simulink model "pfb_fir_2p_2kpt_12i_18o_os2_core"  (R2021a)
(part 3 of 41)

      mask prompts: mult_latency "Multiplier Latency"; coeff_width "Coefficient Bit Width In"; coeff_frac_width "Coefficient Fractional Bits"; delay "Data/Sync Delay"; data_width "Data Bit Width In"; bram_latency "BRAM Latency"; use_hdl "Use behavioral HDL for multlipliers"; use_embedded "Use embedded multipliers"
      mask init: same as pfb_fir_2p_2kpt_12i_18o_os2_core/pfb_fir/pol1_in10_tap2
      mask Callback use_hdl:
      | use_hdl = get_param(gcb,'use_hdl');
      | if( strcmp(use_hdl,'on')),
      |     set_param(gcb, 'use_embedded','off');
      |     set_param(gcb, 'MaskVisibilities',{'on','on','on','on','on','on','on','off'});
      | else,
      |     set_param(gcb, 'MaskVisibilities',{'on','on','on','on','on','on','on','on'});
      | end
  pol1_in8_tap3 : Subsystem  AncestorBlock=casper_library_pfbs/tap  mask(tap){mult_latency=2, coeff_width=18, coeff_frac_width=17, delay=128, data_width=12, bram_latency=2, use_hdl=on, use_embedded=off}
      mask prompts: mult_latency "Multiplier Latency"; coeff_width "Coefficient Bit Width In"; coeff_frac_width "Coefficient Fractional Bits"; delay "Data/Sync Delay"; data_width "Data Bit Width In"; bram_latency "BRAM Latency"; use_hdl "Use behavioral HDL for multlipliers"; use_embedded "Use embedded multipliers"
      mask init: same as pfb_fir_2p_2kpt_12i_18o_os2_core/pfb_fir/pol1_in10_tap2
      mask Callback use_hdl:
      | use_hdl = get_param(gcb,'use_hdl');
      | if( strcmp(use_hdl,'on')),
      |     set_param(gcb, 'use_embedded','off');
      |     set_param(gcb, 'MaskVisibilities',{'on','on','on','on','on','on','on','off'});
      | else,
      |     set_param(gcb, 'MaskVisibilities',{'on','on','on','on','on','on','on','on'});
      | end
  pol1_in8_tap4 : Subsystem  AncestorBlock=casper_library_pfbs/tap  mask(tap){mult_latency=2, coeff_width=18, coeff_frac_width=17, delay=128, data_width=12, bram_latency=2, use_hdl=on, use_embedded=off}
      mask prompts: mult_latency "Multiplier Latency"; coeff_width "Coefficient Bit Width In"; coeff_frac_width "Coefficient Fractional Bits"; delay "Data/Sync Delay"; data_width "Data Bit Width In"; bram_latency "BRAM Latency"; use_hdl "Use behavioral HDL for multlipliers"; use_embedded "Use embedded multipliers"
      mask init: same as pfb_fir_2p_2kpt_12i_18o_os2_core/pfb_fir/pol1_in10_tap2
      mask Callback use_hdl:
      | use_hdl = get_param(gcb,'use_hdl');
      | if( strcmp(use_hdl,'on')),
      |     set_param(gcb, 'use_embedded','off');
      |     set_param(gcb, 'MaskVisibilities',{'on','on','on','on','on','on','on','off'});
      | else,
      |     set_param(gcb, 'MaskVisibilities',{'on','on','on','on','on','on','on','on'});
      | end
  pol1_in8_tap5 : Subsystem  AncestorBlock=casper_library_pfbs/tap  mask(tap){mult_latency=2, coeff_width=18, coeff_frac_width=17, delay=128, data_width=12, bram_latency=2, use_hdl=on, use_embedded=off}
      mask prompts: mult_latency "Multiplier Latency"; coeff_width "Coefficient Bit Width In"; coeff_frac_width "Coefficient Fractional Bits"; delay "Data/Sync Delay"; data_width "Data Bit Width In"; bram_latency "BRAM Latency"; use_hdl "Use behavioral HDL for multlipliers"; use_embedded "Use embedded multipliers"
      mask init: same as pfb_fir_2p_2kpt_12i_18o_os2_core/pfb_fir/pol1_in10_tap2
      mask Callback use_hdl:
      | use_hdl = get_param(gcb,'use_hdl');
      | if( strcmp(use_hdl,'on')),
      |     set_param(gcb, 'use_embedded','off');
      |     set_param(gcb, 'MaskVisibilities',{'on','on','on','on','on','on','on','off'});
      | else,
      |     set_param(gcb, 'MaskVisibilities',{'on','on','on','on','on','on','on','on'});
      | end
  pol1_in8_tap6 : Subsystem  AncestorBlock=casper_library_pfbs/tap  mask(tap){mult_latency=2, coeff_width=18, coeff_frac_width=17, delay=128, data_width=12, bram_latency=2, use_hdl=on, use_embedded=off}
      mask prompts: mult_latency "Multiplier Latency"; coeff_width "Coefficient Bit Width In"; coeff_frac_width "Coefficient Fractional Bits"; delay "Data/Sync Delay"; data_width "Data Bit Width In"; bram_latency "BRAM Latency"; use_hdl "Use behavioral HDL for multlipliers"; use_embedded "Use embedded multipliers"
      mask init: same as pfb_fir_2p_2kpt_12i_18o_os2_core/pfb_fir/pol1_in10_tap2
      mask Callback use_hdl:
      | use_hdl = get_param(gcb,'use_hdl');
      | if( strcmp(use_hdl,'on')),
      |     set_param(gcb, 'use_embedded','off');
      |     set_param(gcb, 'MaskVisibilities',{'on','on','on','on','on','on','on','off'});
      | else,
      |     set_param(gcb, 'MaskVisibilities',{'on','on','on','on','on','on','on','on'});
      | end
  pol1_in8_tap7 : Subsystem  AncestorBlock=casper_library_pfbs/tap  mask(tap){mult_latency=2, coeff_width=18, coeff_frac_width=17, delay=128, data_width=12, bram_latency=2, use_hdl=on, use_embedded=off}
      mask prompts: mult_latency "Multiplier Latency"; coeff_width "Coefficient Bit Width In"; coeff_frac_width "Coefficient Fractional Bits"; delay "Data/Sync Delay"; data_width "Data Bit Width In"; bram_latency "BRAM Latency"; use_hdl "Use behavioral HDL for multlipliers"; use_embedded "Use embedded multipliers"
      mask init: same as pfb_fir_2p_2kpt_12i_18o_os2_core/pfb_fir/pol1_in10_tap2
      mask Callback use_hdl:
      | use_hdl = get_param(gcb,'use_hdl');
      | if( strcmp(use_hdl,'on')),
      |     set_param(gcb, 'use_embedded','off');
      |     set_param(gcb, 'MaskVisibilities',{'on','on','on','on','on','on','on','off'});
      | else,
      |     set_param(gcb, 'MaskVisibilities',{'on','on','on','on','on','on','on','on'});
      | end
  pol1_in9_coeffs : Subsystem  AncestorBlock=casper_library_pfbs/pfb_coeff_gen  mask(pfb_coeff_gen){PFBSize=11, CoeffBitWidth=18, TotalTaps=8, CoeffDistMem=off, WindowType=hamming, bram_latency=2, n_inputs=4, nput=8, fwidth=1, debug_mode=off, fan_latency=1}
      mask prompts: PFBSize "Size of PFB: (2^? pnts)"; CoeffBitWidth "Bitwidth of Coefficients:"; TotalTaps "Total Number of Taps:"; CoeffDistMem "Implement Coeff Gen in Distributed Memory"; WindowType "Windowing Function:"; bram_latency "BRAM Latency"; n_inputs "Number of Simultaneous Inputs: (2^?)"; nput "This is input number:"; fwidth "Bin Width (normal=1)"; debug_mode "Debug mode - coeffs are a [1:pfb_size*taps] ramp."; fan_latency "Fanout latency"
      mask init: same as pfb_fir_2p_2kpt_12i_18o_os2_core/pfb_fir/pol1_in10_coeffs
      settings: AttributesFormatString=|
      | PFBSize=11, n_inputs=4,
      | taps=8, input=8
  pol1_in9_first_tap : Subsystem  AncestorBlock=casper_library_pfbs/first_tap  mask(first_tap){PFBSize=11, n_pol_blocks=1, CoeffBitWidth=18, TotalTaps=8, BitWidthIn=12, WindowType=hamming, mult_latency=2, bram_latency=2, n_inputs=4, fwidth=1, use_hdl=on, use_embedded=off}
      mask prompts: PFBSize "Size of PFB: (2^? pnts)"; n_pol_blocks "Number of serial polarization blocks"; CoeffBitWidth "Bitwidth of Coefficients:"; TotalTaps "Total Number of Taps:"; BitWidthIn "Input Bitwidth:"; WindowType "Windowing Function:"; mult_latency "Mult Latency"; bram_latency "BRAM Latency"; n_inputs "Number of Simultaneous Inputs: (2^?)"; fwidth "Bit Width (normal=1)"; use_hdl "Use behavioral HDL for multlipliers"; use_embedded "Use embedded multipliers"
      mask init: same as pfb_fir_2p_2kpt_12i_18o_os2_core/pfb_fir/pol1_in10_first_tap
      settings: AttributesFormatString=taps=8
      mask TypeOptions WindowType: bartlett | barthannwin | blackman | blackmanharris | bohamwin | chebwin | flattopwin | gausswin | hamming | hann | kaiser | nuttallwin | parzenwin | rectwin | tukeywin | triang
      mask Callback use_hdl:
      | use_hdl = get_param(gcb,'use_hdl');
      | if( strcmp(use_hdl,'on')),
      |     set_param(gcb, 'use_embedded','off');
      |     set_param(gcb, 'MaskVisibilities',{'on','on','on','on','on','on','on','on','on','on','on','off'});
      | else,
      |     set_param(gcb, 'MaskVisibilities',{'on','on','on','on','on','on','on','on','on','on','on','on'});
      | end
  pol1_in9_last_tap : Subsystem  AncestorBlock=casper_library_pfbs/last_tap_oversample2x  mask(last_tap_oversample2x){TotalTaps=8, BitWidthIn=12, BitWidthOut=18, CoeffBitWidth=18, add_latency=1, mult_latency=2, quantization=Round  (unbiased: Even Values), use_hdl=on, use_embedded=off}
      mask prompts: TotalTaps "Total Number of Taps:"; BitWidthIn "Input Bitwidth:"; BitWidthOut "Output Bitwidth:"; CoeffBitWidth "Coeff Bitwidth:"; add_latency "Add Latency"; mult_latency "Mult Latency"; quantization "Quantization Behavior"; use_hdl "Use behavioral HDL for multlipliers"; use_embedded "Use embedded multipliers"
      mask init: same as pfb_fir_2p_2kpt_12i_18o_os2_core/pfb_fir/pol1_in10_last_tap
      settings: AttributesFormatString=taps=8
      mask TypeOptions quantization: Truncate | Round  (unbiased: +/- Inf) | Round  (unbiased: Even Values)
      mask Callback use_hdl:
      | use_hdl = get_param(gcb,'use_hdl');
      | if( strcmp(use_hdl,'on')),
      |     set_param(gcb, 'use_embedded','off');
      |     set_param(gcb, 'MaskVisibilities',{'on','on','on','on','on','on','on','on','off'});
      | else,
      |     set_param(gcb, 'MaskVisibilities',{'on','on','on','on','on','on','on','on','on'});
      | end
  pol1_in9_tap2 : Subsystem  AncestorBlock=casper_library_pfbs/tap  mask(tap){mult_latency=2, coeff_width=18, coeff_frac_width=17, delay=128, data_width=12, bram_latency=2, use_hdl=on, use_embedded=off}
      mask prompts: mult_latency "Multiplier Latency"; coeff_width "Coefficient Bit Width In"; coeff_frac_width "Coefficient Fractional Bits"; delay "Data/Sync Delay"; data_width "Data Bit Width In"; bram_latency "BRAM Latency"; use_hdl "Use behavioral HDL for multlipliers"; use_embedded "Use embedded multipliers"
      mask init: same as pfb_fir_2p_2kpt_12i_18o_os2_core/pfb_fir/pol1_in10_tap2
      mask Callback use_hdl:
      | use_hdl = get_param(gcb,'use_hdl');
      | if( strcmp(use_hdl,'on')),
      |     set_param(gcb, 'use_embedded','off');
      |     set_param(gcb, 'MaskVisibilities',{'on','on','on','on','on','on','on','off'});
      | else,
      |     set_param(gcb, 'MaskVisibilities',{'on','on','on','on','on','on','on','on'});
      | end
  pol1_in9_tap3 : Subsystem  AncestorBlock=casper_library_pfbs/tap  mask(tap){mult_latency=2, coeff_width=18, coeff_frac_width=17, delay=128, data_width=12, bram_latency=2, use_hdl=on, use_embedded=off}
      mask prompts: mult_latency "Multiplier Latency"; coeff_width "Coefficient Bit Width In"; coeff_frac_width "Coefficient Fractional Bits"; delay "Data/Sync Delay"; data_width "Data Bit Width In"; bram_latency "BRAM Latency"; use_hdl "Use behavioral HDL for multlipliers"; use_embedded "Use embedded multipliers"
      mask init: same as pfb_fir_2p_2kpt_12i_18o_os2_core/pfb_fir/pol1_in10_tap2
      mask Callback use_hdl:
      | use_hdl = get_param(gcb,'use_hdl');
      | if( strcmp(use_hdl,'on')),
      |     set_param(gcb, 'use_embedded','off');
      |     set_param(gcb, 'MaskVisibilities',{'on','on','on','on','on','on','on','off'});
      | else,
      |     set_param(gcb, 'MaskVisibilities',{'on','on','on','on','on','on','on','on'});
      | end
  pol1_in9_tap4 : Subsystem  AncestorBlock=casper_library_pfbs/tap  mask(tap){mult_latency=2, coeff_width=18, coeff_frac_width=17, delay=128, data_width=12, bram_latency=2, use_hdl=on, use_embedded=off}
      mask prompts: mult_latency "Multiplier Latency"; coeff_width "Coefficient Bit Width In"; coeff_frac_width "Coefficient Fractional Bits"; delay "Data/Sync Delay"; data_width "Data Bit Width In"; bram_latency "BRAM Latency"; use_hdl "Use behavioral HDL for multlipliers"; use_embedded "Use embedded multipliers"
      mask init: same as pfb_fir_2p_2kpt_12i_18o_os2_core/pfb_fir/pol1_in10_tap2
      mask Callback use_hdl:
      | use_hdl = get_param(gcb,'use_hdl');
      | if( strcmp(use_hdl,'on')),
      |     set_param(gcb, 'use_embedded','off');
      |     set_param(gcb, 'MaskVisibilities',{'on','on','on','on','on','on','on','off'});
      | else,
      |     set_param(gcb, 'MaskVisibilities',{'on','on','on','on','on','on','on','on'});
      | end
  pol1_in9_tap5 : Subsystem  AncestorBlock=casper_library_pfbs/tap  mask(tap){mult_latency=2, coeff_width=18, coeff_frac_width=17, delay=128, data_width=12, bram_latency=2, use_hdl=on, use_embedded=off}
      mask prompts: mult_latency "Multiplier Latency"; coeff_width "Coefficient Bit Width In"; coeff_frac_width "Coefficient Fractional Bits"; delay "Data/Sync Delay"; data_width "Data Bit Width In"; bram_latency "BRAM Latency"; use_hdl "Use behavioral HDL for multlipliers"; use_embedded "Use embedded multipliers"
      mask init: same as pfb_fir_2p_2kpt_12i_18o_os2_core/pfb_fir/pol1_in10_tap2
      mask Callback use_hdl:
      | use_hdl = get_param(gcb,'use_hdl');
      | if( strcmp(use_hdl,'on')),
      |     set_param(gcb, 'use_embedded','off');
      |     set_param(gcb, 'MaskVisibilities',{'on','on','on','on','on','on','on','off'});
      | else,
      |     set_param(gcb, 'MaskVisibilities',{'on','on','on','on','on','on','on','on'});
      | end
  pol1_in9_tap6 : Subsystem  AncestorBlock=casper_library_pfbs/tap  mask(tap){mult_latency=2, coeff_width=18, coeff_frac_width=17, delay=128, data_width=12, bram_latency=2, use_hdl=on, use_embedded=off}
      mask prompts: mult_latency "Multiplier Latency"; coeff_width "Coefficient Bit Width In"; coeff_frac_width "Coefficient Fractional Bits"; delay "Data/Sync Delay"; data_width "Data Bit Width In"; bram_latency "BRAM Latency"; use_hdl "Use behavioral HDL for multlipliers"; use_embedded "Use embedded multipliers"
      mask init: same as pfb_fir_2p_2kpt_12i_18o_os2_core/pfb_fir/pol1_in10_tap2
      mask Callback use_hdl:
      | use_hdl = get_param(gcb,'use_hdl');
      | if( strcmp(use_hdl,'on')),
      |     set_param(gcb, 'use_embedded','off');
      |     set_param(gcb, 'MaskVisibilities',{'on','on','on','on','on','on','on','off'});
      | else,
      |     set_param(gcb, 'MaskVisibilities',{'on','on','on','on','on','on','on','on'});
      | end
  pol1_in9_tap7 : Subsystem  AncestorBlock=casper_library_pfbs/tap  mask(tap){mult_latency=2, coeff_width=18, coeff_frac_width=17, delay=128, data_width=12, bram_latency=2, use_hdl=on, use_embedded=off}
      mask prompts: mult_latency "Multiplier Latency"; coeff_width "Coefficient Bit Width In"; coeff_frac_width "Coefficient Fractional Bits"; delay "Data/Sync Delay"; data_width "Data Bit Width In"; bram_latency "BRAM Latency"; use_hdl "Use behavioral HDL for multlipliers"; use_embedded "Use embedded multipliers"
      mask init: same as pfb_fir_2p_2kpt_12i_18o_os2_core/pfb_fir/pol1_in10_tap2
      mask Callback use_hdl:
      | use_hdl = get_param(gcb,'use_hdl');
      | if( strcmp(use_hdl,'on')),
      |     set_param(gcb, 'use_embedded','off');
      |     set_param(gcb, 'MaskVisibilities',{'on','on','on','on','on','on','on','off'});
      | else,
      |     set_param(gcb, 'MaskVisibilities',{'on','on','on','on','on','on','on','on'});
      | end
  pol1_in_bus_create1 : Subsystem  AncestorBlock=casper_library_flow_control/bus_create  mask(bus_create){inputNum=16}
      mask prompts: inputNum "Number of inputs:"
      mask init:
      | bus_create_init(gcb,...
      |     'inputNum', inputNum);
  pol1_in_bus_create2 : Subsystem  AncestorBlock=casper_library_flow_control/bus_create  mask(bus_create){inputNum=16}
      mask prompts: inputNum "Number of inputs:"
      mask init:
      | bus_create_init(gcb,...
      |     'inputNum', inputNum);
  pol1_reord : Subsystem  AncestorBlock=casper_library_reorder/reorder  mask(reorder){map=reshape(transpose(reshape([0:127], 2, 64)), 128, 1), n_bits=0, n_inputs=1, bram_latency=3, map_latency=1, fanout_latency=0, double_buffer=0, bram_map=off, software_controlled=off}
      mask prompts: map "Output Order:"; n_bits "Data width in"; n_inputs "Number of inputs"; bram_latency "BRAM Latency"; map_latency "Map Latency"; fanout_latency "Fanout latency"; double_buffer "Double Buffer"; bram_map "Use BlockRAM for Map"; software_controlled "Use runtime software control"
      mask init:
      | reorder_init(gcb, ...
      |     'map', map, ...
      |     'n_bits', n_bits, ...
      |     'n_inputs', n_inputs, ...
      |     'bram_latency', bram_latency, ...
      |     'map_latency', map_latency, ...
      |     'fanout_latency', fanout_latency, ...
      |     'double_buffer', double_buffer, ...
      |     'bram_map', bram_map, ...
      |     'software_controlled', software_controlled);
      settings: AttributesFormatString=order=7
      mask Help: eval('xlWeb(''http://casper.berkeley.edu/wiki/Reorder'')')
  pol1_reord_in_bus_create : Subsystem  AncestorBlock=casper_library_flow_control/bus_create  mask(bus_create){inputNum=2}
      mask prompts: inputNum "Number of inputs:"
      mask init:
      | bus_create_init(gcb,...
      |     'inputNum', inputNum);
  pol1_transpose : Subsystem  AncestorBlock=casper_library_reorder/square_transposer  mask(square_transposer){n_inputs=1, async=off}
      mask prompts: n_inputs "Number of inputs (2^?):"; async "Aynchronus operation"
      mask init:
      | square_transposer_init(gcb,...
      |     'n_inputs', n_inputs, ...
      |     'async', async);
      settings: AttributesFormatString=n_inputs=1
      mask Help: eval('xlWeb(''http://casper.berkeley.edu/wiki/Square_transposer'')')
  sync_out : Outport  VectorParamsAs1DForOutWhenUnconnected=off
  pol1_out1 : Outport  Port=2  VectorParamsAs1DForOutWhenUnconnected=off
  pol1_out2 : Outport  Port=3  VectorParamsAs1DForOutWhenUnconnected=off
  pol1_out3 : Outport  Port=4
  pol1_out4 : Outport  Port=5
  pol1_out5 : Outport  Port=6
  pol1_out6 : Outport  Port=7
  pol1_out7 : Outport  Port=8
  pol1_out8 : Outport  Port=9
  pol1_out9 : Outport  Port=10
  pol1_out10 : Outport  Port=11
  pol1_out11 : Outport  Port=12
  pol1_out12 : Outport  Port=13
  pol1_out13 : Outport  Port=14
  pol1_out14 : Outport  Port=15
  pol1_out15 : Outport  Port=16
  pol1_out16 : Outport  Port=17
  pol1_out17 : Outport  Port=18
  pol1_out18 : Outport  Port=19
  pol1_out19 : Outport  Port=20
  pol1_out20 : Outport  Port=21
  pol1_out21 : Outport  Port=22
  pol1_out22 : Outport  Port=23
  pol1_out23 : Outport  Port=24
  pol1_out24 : Outport  Port=25
  pol1_out25 : Outport  Port=26
  pol1_out26 : Outport  Port=27
  pol1_out27 : Outport  Port=28
  pol1_out28 : Outport  Port=29
  pol1_out29 : Outport  Port=30
  pol1_out30 : Outport  Port=31
  pol1_out31 : Outport  Port=32
  pol1_out32 : Outport  Port=33
  wires:
  pol1_in1/1 -> pol1_in1_coeffs/1(din)
  sync/1 -> pol1_in1_coeffs/2(sync), pol1_in2_coeffs/2(sync), pol1_in3_coeffs/2(sync), pol1_in4_coeffs/2(sync), pol1_in5_coeffs/2(sync), pol1_in6_coeffs/2(sync), pol1_in7_coeffs/2(sync), pol1_in8_coeffs/2(sync), pol1_in9_coeffs/2(sync), pol1_in10_coeffs/2(sync), pol1_in11_coeffs/2(sync), pol1_in12_coeffs/2(sync), pol1_in13_coeffs/2(sync), pol1_in14_coeffs/2(sync), pol1_in15_coeffs/2(sync), pol1_in16_coeffs/2(sync)
  pol1_in1_coeffs/1(dout) -> pol1_in1_first_tap/1(din)
  pol1_in1_coeffs/2(sync_out) -> pol1_in1_first_tap/2(sync), pol1_in2_first_tap/2(sync), pol1_in3_first_tap/2(sync), pol1_in4_first_tap/2(sync), pol1_in5_first_tap/2(sync), pol1_in6_first_tap/2(sync), pol1_in7_first_tap/2(sync), pol1_in8_first_tap/2(sync), pol1_in9_first_tap/2(sync), pol1_in10_first_tap/2(sync), pol1_in11_first_tap/2(sync), pol1_in12_first_tap/2(sync), pol1_in13_first_tap/2(sync), pol1_in14_first_tap/2(sync), pol1_in15_first_tap/2(sync), pol1_in16_first_tap/2(sync)
  pol1_in1_coeffs/3(coeff) -> pol1_in1_first_tap/3(coeffs)
  pol1_in1_first_tap/1(dout) -> pol1_in1_tap2/1(din)
  pol1_in1_first_tap/2(sync_out) -> pol1_in1_tap2/2(sync)
  pol1_in1_first_tap/3(coeff_out) -> pol1_in1_tap2/3(coeff)
  pol1_in1_first_tap/4(taps_out) -> pol1_in1_tap2/4(taps)
  pol1_in1_tap2/1(dout) -> pol1_in1_tap3/1(din)
  pol1_in1_tap2/2(sync_out) -> pol1_in1_tap3/2(sync)
  pol1_in1_tap2/3(coeff_out) -> pol1_in1_tap3/3(coeff)
  pol1_in1_tap2/4(taps_out) -> pol1_in1_tap3/4(taps)
  pol1_in1_tap3/1(dout) -> pol1_in1_tap4/1(din)
  pol1_in1_tap3/2(sync_out) -> pol1_in1_tap4/2(sync)
  pol1_in1_tap3/3(coeff_out) -> pol1_in1_tap4/3(coeff)
  pol1_in1_tap3/4(taps_out) -> pol1_in1_tap4/4(taps)
  pol1_in1_tap4/1(dout) -> pol1_in1_tap5/1(din)
  pol1_in1_tap4/2(sync_out) -> pol1_in1_tap5/2(sync)
  pol1_in1_tap4/3(coeff_out) -> pol1_in1_tap5/3(coeff)
  pol1_in1_tap4/4(taps_out) -> pol1_in1_tap5/4(taps)
  pol1_in1_tap5/1(dout) -> pol1_in1_tap6/1(din)
  pol1_in1_tap5/2(sync_out) -> pol1_in1_tap6/2(sync)
  pol1_in1_tap5/3(coeff_out) -> pol1_in1_tap6/3(coeff)
  pol1_in1_tap5/4(taps_out) -> pol1_in1_tap6/4(taps)
  pol1_in1_tap6/1(dout) -> pol1_in1_tap7/1(din)
  pol1_in1_tap6/2(sync_out) -> pol1_in1_tap7/2(sync)
  pol1_in1_tap6/3(coeff_out) -> pol1_in1_tap7/3(coeff)
  pol1_in1_tap6/4(taps_out) -> pol1_in1_tap7/4(taps)
  pol1_in1_tap7/1(dout) -> pol1_in1_last_tap/1(din)
  pol1_in1_tap7/2(sync_out) -> pol1_in1_last_tap/2(sync)
  pol1_in1_tap7/3(coeff_out) -> pol1_in1_last_tap/3(coeff)
  pol1_in1_tap7/4(taps_out) -> pol1_in1_last_tap/4(taps)
  pol1_in2/1 -> pol1_in2_coeffs/1(din)
  pol1_in2_coeffs/1(dout) -> pol1_in2_first_tap/1(din)
  pol1_in2_coeffs/3(coeff) -> pol1_in2_first_tap/3(coeffs)
  pol1_in2_first_tap/1(dout) -> pol1_in2_tap2/1(din)
  pol1_in2_first_tap/2(sync_out) -> pol1_in2_tap2/2(sync)
  pol1_in2_first_tap/3(coeff_out) -> pol1_in2_tap2/3(coeff)
  pol1_in2_first_tap/4(taps_out) -> pol1_in2_tap2/4(taps)
  pol1_in2_tap2/1(dout) -> pol1_in2_tap3/1(din)
  pol1_in2_tap2/2(sync_out) -> pol1_in2_tap3/2(sync)
  pol1_in2_tap2/3(coeff_out) -> pol1_in2_tap3/3(coeff)
  pol1_in2_tap2/4(taps_out) -> pol1_in2_tap3/4(taps)
  pol1_in2_tap3/1(dout) -> pol1_in2_tap4/1(din)
  pol1_in2_tap3/2(sync_out) -> pol1_in2_tap4/2(sync)
  pol1_in2_tap3/3(coeff_out) -> pol1_in2_tap4/3(coeff)
  pol1_in2_tap3/4(taps_out) -> pol1_in2_tap4/4(taps)
  pol1_in2_tap4/1(dout) -> pol1_in2_tap5/1(din)
  pol1_in2_tap4/2(sync_out) -> pol1_in2_tap5/2(sync)
  pol1_in2_tap4/3(coeff_out) -> pol1_in2_tap5/3(coeff)
  pol1_in2_tap4/4(taps_out) -> pol1_in2_tap5/4(taps)
  pol1_in2_tap5/1(dout) -> pol1_in2_tap6/1(din)
  pol1_in2_tap5/2(sync_out) -> pol1_in2_tap6/2(sync)
  pol1_in2_tap5/3(coeff_out) -> pol1_in2_tap6/3(coeff)
  pol1_in2_tap5/4(taps_out) -> pol1_in2_tap6/4(taps)
  pol1_in2_tap6/1(dout) -> pol1_in2_tap7/1(din)
  pol1_in2_tap6/2(sync_out) -> pol1_in2_tap7/2(sync)
  pol1_in2_tap6/3(coeff_out) -> pol1_in2_tap7/3(coeff)
  pol1_in2_tap6/4(taps_out) -> pol1_in2_tap7/4(taps)
  pol1_in2_tap7/1(dout) -> pol1_in2_last_tap/1(din)
  pol1_in2_tap7/2(sync_out) -> pol1_in2_last_tap/2(sync)
  pol1_in2_tap7/3(coeff_out) -> pol1_in2_last_tap/3(coeff)
  pol1_in2_tap7/4(taps_out) -> pol1_in2_last_tap/4(taps)
  pol1_in3/1 -> pol1_in3_coeffs/1(din)
  pol1_in3_coeffs/1(dout) -> pol1_in3_first_tap/1(din)
  pol1_in3_coeffs/3(coeff) -> pol1_in3_first_tap/3(coeffs)
  pol1_in3_first_tap/1(dout) -> pol1_in3_tap2/1(din)
  pol1_in3_first_tap/2(sync_out) -> pol1_in3_tap2/2(sync)
  pol1_in3_first_tap/3(coeff_out) -> pol1_in3_tap2/3(coeff)
  pol1_in3_first_tap/4(taps_out) -> pol1_in3_tap2/4(taps)
  pol1_in3_tap2/1(dout) -> pol1_in3_tap3/1(din)
  pol1_in3_tap2/2(sync_out) -> pol1_in3_tap3/2(sync)
  pol1_in3_tap2/3(coeff_out) -> pol1_in3_tap3/3(coeff)
  pol1_in3_tap2/4(taps_out) -> pol1_in3_tap3/4(taps)
  pol1_in3_tap3/1(dout) -> pol1_in3_tap4/1(din)
  pol1_in3_tap3/2(sync_out) -> pol1_in3_tap4/2(sync)
  pol1_in3_tap3/3(coeff_out) -> pol1_in3_tap4/3(coeff)
  pol1_in3_tap3/4(taps_out) -> pol1_in3_tap4/4(taps)
  pol1_in3_tap4/1(dout) -> pol1_in3_tap5/1(din)
  pol1_in3_tap4/2(sync_out) -> pol1_in3_tap5/2(sync)
  pol1_in3_tap4/3(coeff_out) -> pol1_in3_tap5/3(coeff)
  pol1_in3_tap4/4(taps_out) -> pol1_in3_tap5/4(taps)
  pol1_in3_tap5/1(dout) -> pol1_in3_tap6/1(din)
  pol1_in3_tap5/2(sync_out) -> pol1_in3_tap6/2(sync)
  pol1_in3_tap5/3(coeff_out) -> pol1_in3_tap6/3(coeff)
  pol1_in3_tap5/4(taps_out) -> pol1_in3_tap6/4(taps)
  pol1_in3_tap6/1(dout) -> pol1_in3_tap7/1(din)
  pol1_in3_tap6/2(sync_out) -> pol1_in3_tap7/2(sync)
  pol1_in3_tap6/3(coeff_out) -> pol1_in3_tap7/3(coeff)
  pol1_in3_tap6/4(taps_out) -> pol1_in3_tap7/4(taps)
  pol1_in3_tap7/1(dout) -> pol1_in3_last_tap/1(din)
  pol1_in3_tap7/2(sync_out) -> pol1_in3_last_tap/2(sync)
  pol1_in3_tap7/3(coeff_out) -> pol1_in3_last_tap/3(coeff)
  pol1_in3_tap7/4(taps_out) -> pol1_in3_last_tap/4(taps)
  pol1_in4/1 -> pol1_in4_coeffs/1(din)
  pol1_in4_coeffs/1(dout) -> pol1_in4_first_tap/1(din)
  pol1_in4_coeffs/3(coeff) -> pol1_in4_first_tap/3(coeffs)
  pol1_in4_first_tap/1(dout) -> pol1_in4_tap2/1(din)
  pol1_in4_first_tap/2(sync_out) -> pol1_in4_tap2/2(sync)
  pol1_in4_first_tap/3(coeff_out) -> pol1_in4_tap2/3(coeff)
  pol1_in4_first_tap/4(taps_out) -> pol1_in4_tap2/4(taps)
  pol1_in4_tap2/1(dout) -> pol1_in4_tap3/1(din)
  pol1_in4_tap2/2(sync_out) -> pol1_in4_tap3/2(sync)
  pol1_in4_tap2/3(coeff_out) -> pol1_in4_tap3/3(coeff)
  pol1_in4_tap2/4(taps_out) -> pol1_in4_tap3/4(taps)
  pol1_in4_tap3/1(dout) -> pol1_in4_tap4/1(din)
  pol1_in4_tap3/2(sync_out) -> pol1_in4_tap4/2(sync)
  pol1_in4_tap3/3(coeff_out) -> pol1_in4_tap4/3(coeff)
  pol1_in4_tap3/4(taps_out) -> pol1_in4_tap4/4(taps)
  pol1_in4_tap4/1(dout) -> pol1_in4_tap5/1(din)
  pol1_in4_tap4/2(sync_out) -> pol1_in4_tap5/2(sync)
  pol1_in4_tap4/3(coeff_out) -> pol1_in4_tap5/3(coeff)
  pol1_in4_tap4/4(taps_out) -> pol1_in4_tap5/4(taps)
  pol1_in4_tap5/1(dout) -> pol1_in4_tap6/1(din)
  pol1_in4_tap5/2(sync_out) -> pol1_in4_tap6/2(sync)
  pol1_in4_tap5/3(coeff_out) -> pol1_in4_tap6/3(coeff)
  pol1_in4_tap5/4(taps_out) -> pol1_in4_tap6/4(taps)
  pol1_in4_tap6/1(dout) -> pol1_in4_tap7/1(din)
  pol1_in4_tap6/2(sync_out) -> pol1_in4_tap7/2(sync)
  pol1_in4_tap6/3(coeff_out) -> pol1_in4_tap7/3(coeff)
  pol1_in4_tap6/4(taps_out) -> pol1_in4_tap7/4(taps)
  pol1_in4_tap7/1(dout) -> pol1_in4_last_tap/1(din)
  pol1_in4_tap7/2(sync_out) -> pol1_in4_last_tap/2(sync)
  pol1_in4_tap7/3(coeff_out) -> pol1_in4_last_tap/3(coeff)
  pol1_in4_tap7/4(taps_out) -> pol1_in4_last_tap/4(taps)
  pol1_in5/1 -> pol1_in5_coeffs/1(din)
  pol1_in5_coeffs/1(dout) -> pol1_in5_first_tap/1(din)
  pol1_in5_coeffs/3(coeff) -> pol1_in5_first_tap/3(coeffs)
  pol1_in5_first_tap/1(dout) -> pol1_in5_tap2/1(din)
  pol1_in5_first_tap/2(sync_out) -> pol1_in5_tap2/2(sync)
  pol1_in5_first_tap/3(coeff_out) -> pol1_in5_tap2/3(coeff)
  pol1_in5_first_tap/4(taps_out) -> pol1_in5_tap2/4(taps)
  pol1_in5_tap2/1(dout) -> pol1_in5_tap3/1(din)
  pol1_in5_tap2/2(sync_out) -> pol1_in5_tap3/2(sync)
  pol1_in5_tap2/3(coeff_out) -> pol1_in5_tap3/3(coeff)
  pol1_in5_tap2/4(taps_out) -> pol1_in5_tap3/4(taps)
  pol1_in5_tap3/1(dout) -> pol1_in5_tap4/1(din)
  pol1_in5_tap3/2(sync_out) -> pol1_in5_tap4/2(sync)
  pol1_in5_tap3/3(coeff_out) -> pol1_in5_tap4/3(coeff)
  pol1_in5_tap3/4(taps_out) -> pol1_in5_tap4/4(taps)
  pol1_in5_tap4/1(dout) -> pol1_in5_tap5/1(din)
  pol1_in5_tap4/2(sync_out) -> pol1_in5_tap5/2(sync)
  pol1_in5_tap4/3(coeff_out) -> pol1_in5_tap5/3(coeff)
  pol1_in5_tap4/4(taps_out) -> pol1_in5_tap5/4(taps)
  pol1_in5_tap5/1(dout) -> pol1_in5_tap6/1(din)
  pol1_in5_tap5/2(sync_out) -> pol1_in5_tap6/2(sync)
  pol1_in5_tap5/3(coeff_out) -> pol1_in5_tap6/3(coeff)
  pol1_in5_tap5/4(taps_out) -> pol1_in5_tap6/4(taps)
  pol1_in5_tap6/1(dout) -> pol1_in5_tap7/1(din)
  pol1_in5_tap6/2(sync_out) -> pol1_in5_tap7/2(sync)
  pol1_in5_tap6/3(coeff_out) -> pol1_in5_tap7/3(coeff)
  pol1_in5_tap6/4(taps_out) -> pol1_in5_tap7/4(taps)
  pol1_in5_tap7/1(dout) -> pol1_in5_last_tap/1(din)
  pol1_in5_tap7/2(sync_out) -> pol1_in5_last_tap/2(sync)
  pol1_in5_tap7/3(coeff_out) -> pol1_in5_last_tap/3(coeff)
  pol1_in5_tap7/4(taps_out) -> pol1_in5_last_tap/4(taps)
  pol1_in6/1 -> pol1_in6_coeffs/1(din)
  pol1_in6_coeffs/1(dout) -> pol1_in6_first_tap/1(din)
  pol1_in6_coeffs/3(coeff) -> pol1_in6_first_tap/3(coeffs)
  pol1_in6_first_tap/1(dout) -> pol1_in6_tap2/1(din)
  pol1_in6_first_tap/2(sync_out) -> pol1_in6_tap2/2(sync)
  pol1_in6_first_tap/3(coeff_out) -> pol1_in6_tap2/3(coeff)
  pol1_in6_first_tap/4(taps_out) -> pol1_in6_tap2/4(taps)
  pol1_in6_tap2/1(dout) -> pol1_in6_tap3/1(din)
  pol1_in6_tap2/2(sync_out) -> pol1_in6_tap3/2(sync)
  pol1_in6_tap2/3(coeff_out) -> pol1_in6_tap3/3(coeff)
  pol1_in6_tap2/4(taps_out) -> pol1_in6_tap3/4(taps)
  pol1_in6_tap3/1(dout) -> pol1_in6_tap4/1(din)
  pol1_in6_tap3/2(sync_out) -> pol1_in6_tap4/2(sync)
  pol1_in6_tap3/3(coeff_out) -> pol1_in6_tap4/3(coeff)
  pol1_in6_tap3/4(taps_out) -> pol1_in6_tap4/4(taps)
  pol1_in6_tap4/1(dout) -> pol1_in6_tap5/1(din)
  pol1_in6_tap4/2(sync_out) -> pol1_in6_tap5/2(sync)
  pol1_in6_tap4/3(coeff_out) -> pol1_in6_tap5/3(coeff)
  pol1_in6_tap4/4(taps_out) -> pol1_in6_tap5/4(taps)
  pol1_in6_tap5/1(dout) -> pol1_in6_tap6/1(din)
  pol1_in6_tap5/2(sync_out) -> pol1_in6_tap6/2(sync)
  pol1_in6_tap5/3(coeff_out) -> pol1_in6_tap6/3(coeff)
  pol1_in6_tap5/4(taps_out) -> pol1_in6_tap6/4(taps)
  pol1_in6_tap6/1(dout) -> pol1_in6_tap7/1(din)
  pol1_in6_tap6/2(sync_out) -> pol1_in6_tap7/2(sync)
  pol1_in6_tap6/3(coeff_out) -> pol1_in6_tap7/3(coeff)
  pol1_in6_tap6/4(taps_out) -> pol1_in6_tap7/4(taps)
  pol1_in6_tap7/1(dout) -> pol1_in6_last_tap/1(din)
  pol1_in6_tap7/2(sync_out) -> pol1_in6_last_tap/2(sync)
  pol1_in6_tap7/3(coeff_out) -> pol1_in6_last_tap/3(coeff)
  pol1_in6_tap7/4(taps_out) -> pol1_in6_last_tap/4(taps)
  pol1_in7/1 -> pol1_in7_coeffs/1(din)
  pol1_in7_coeffs/1(dout) -> pol1_in7_first_tap/1(din)
  pol1_in7_coeffs/3(coeff) -> pol1_in7_first_tap/3(coeffs)
  pol1_in7_first_tap/1(dout) -> pol1_in7_tap2/1(din)
  pol1_in7_first_tap/2(sync_out) -> pol1_in7_tap2/2(sync)
  pol1_in7_first_tap/3(coeff_out) -> pol1_in7_tap2/3(coeff)
  pol1_in7_first_tap/4(taps_out) -> pol1_in7_tap2/4(taps)
  pol1_in7_tap2/1(dout) -> pol1_in7_tap3/1(din)
  pol1_in7_tap2/2(sync_out) -> pol1_in7_tap3/2(sync)
  pol1_in7_tap2/3(coeff_out) -> pol1_in7_tap3/3(coeff)
  pol1_in7_tap2/4(taps_out) -> pol1_in7_tap3/4(taps)
  pol1_in7_tap3/1(dout) -> pol1_in7_tap4/1(din)
  pol1_in7_tap3/2(sync_out) -> pol1_in7_tap4/2(sync)
  pol1_in7_tap3/3(coeff_out) -> pol1_in7_tap4/3(coeff)
  pol1_in7_tap3/4(taps_out) -> pol1_in7_tap4/4(taps)
  pol1_in7_tap4/1(dout) -> pol1_in7_tap5/1(din)
  pol1_in7_tap4/2(sync_out) -> pol1_in7_tap5/2(sync)
  pol1_in7_tap4/3(coeff_out) -> pol1_in7_tap5/3(coeff)
  pol1_in7_tap4/4(taps_out) -> pol1_in7_tap5/4(taps)
  pol1_in7_tap5/1(dout) -> pol1_in7_tap6/1(din)
  pol1_in7_tap5/2(sync_out) -> pol1_in7_tap6/2(sync)
  pol1_in7_tap5/3(coeff_out) -> pol1_in7_tap6/3(coeff)
  pol1_in7_tap5/4(taps_out) -> pol1_in7_tap6/4(taps)
  pol1_in7_tap6/1(dout) -> pol1_in7_tap7/1(din)
  pol1_in7_tap6/2(sync_out) -> pol1_in7_tap7/2(sync)
  pol1_in7_tap6/3(coeff_out) -> pol1_in7_tap7/3(coeff)
  pol1_in7_tap6/4(taps_out) -> pol1_in7_tap7/4(taps)
  pol1_in7_tap7/1(dout) -> pol1_in7_last_tap/1(din)
  pol1_in7_tap7/2(sync_out) -> pol1_in7_last_tap/2(sync)
  pol1_in7_tap7/3(coeff_out) -> pol1_in7_last_tap/3(coeff)
  pol1_in7_tap7/4(taps_out) -> pol1_in7_last_tap/4(taps)
  pol1_in8/1 -> pol1_in8_coeffs/1(din)
  pol1_in8_coeffs/1(dout) -> pol1_in8_first_tap/1(din)
  pol1_in8_coeffs/3(coeff) -> pol1_in8_first_tap/3(coeffs)
  pol1_in8_first_tap/1(dout) -> pol1_in8_tap2/1(din)
  pol1_in8_first_tap/2(sync_out) -> pol1_in8_tap2/2(sync)
  pol1_in8_first_tap/3(coeff_out) -> pol1_in8_tap2/3(coeff)
  pol1_in8_first_tap/4(taps_out) -> pol1_in8_tap2/4(taps)
  pol1_in8_tap2/1(dout) -> pol1_in8_tap3/1(din)
  pol1_in8_tap2/2(sync_out) -> pol1_in8_tap3/2(sync)
  pol1_in8_tap2/3(coeff_out) -> pol1_in8_tap3/3(coeff)
  pol1_in8_tap2/4(taps_out) -> pol1_in8_tap3/4(taps)
  pol1_in8_tap3/1(dout) -> pol1_in8_tap4/1(din)
  pol1_in8_tap3/2(sync_out) -> pol1_in8_tap4/2(sync)
  pol1_in8_tap3/3(coeff_out) -> pol1_in8_tap4/3(coeff)
  pol1_in8_tap3/4(taps_out) -> pol1_in8_tap4/4(taps)
  pol1_in8_tap4/1(dout) -> pol1_in8_tap5/1(din)
  pol1_in8_tap4/2(sync_out) -> pol1_in8_tap5/2(sync)
  pol1_in8_tap4/3(coeff_out) -> pol1_in8_tap5/3(coeff)
  pol1_in8_tap4/4(taps_out) -> pol1_in8_tap5/4(taps)
  pol1_in8_tap5/1(dout) -> pol1_in8_tap6/1(din)
  pol1_in8_tap5/2(sync_out) -> pol1_in8_tap6/2(sync)
  pol1_in8_tap5/3(coeff_out) -> pol1_in8_tap6/3(coeff)
  pol1_in8_tap5/4(taps_out) -> pol1_in8_tap6/4(taps)
  pol1_in8_tap6/1(dout) -> pol1_in8_tap7/1(din)
  pol1_in8_tap6/2(sync_out) -> pol1_in8_tap7/2(sync)
  pol1_in8_tap6/3(coeff_out) -> pol1_in8_tap7/3(coeff)
  pol1_in8_tap6/4(taps_out) -> pol1_in8_tap7/4(taps)
  pol1_in8_tap7/1(dout) -> pol1_in8_last_tap/1(din)
  pol1_in8_tap7/2(sync_out) -> pol1_in8_last_tap/2(sync)
  pol1_in8_tap7/3(coeff_out) -> pol1_in8_last_tap/3(coeff)
  pol1_in8_tap7/4(taps_out) -> pol1_in8_last_tap/4(taps)
  pol1_in9/1 -> pol1_in9_coeffs/1(din)
  pol1_in9_coeffs/1(dout) -> pol1_in9_first_tap/1(din)
  pol1_in9_coeffs/3(coeff) -> pol1_in9_first_tap/3(coeffs)
  pol1_in9_first_tap/1(dout) -> pol1_in9_tap2/1(din)
  pol1_in9_first_tap/2(sync_out) -> pol1_in9_tap2/2(sync)
  pol1_in9_first_tap/3(coeff_out) -> pol1_in9_tap2/3(coeff)
  pol1_in9_first_tap/4(taps_out) -> pol1_in9_tap2/4(taps)
  pol1_in9_tap2/1(dout) -> pol1_in9_tap3/1(din)
  pol1_in9_tap2/2(sync_out) -> pol1_in9_tap3/2(sync)
  pol1_in9_tap2/3(coeff_out) -> pol1_in9_tap3/3(coeff)
  pol1_in9_tap2/4(taps_out) -> pol1_in9_tap3/4(taps)
  pol1_in9_tap3/1(dout) -> pol1_in9_tap4/1(din)
  pol1_in9_tap3/2(sync_out) -> pol1_in9_tap4/2(sync)
  pol1_in9_tap3/3(coeff_out) -> pol1_in9_tap4/3(coeff)
  pol1_in9_tap3/4(taps_out) -> pol1_in9_tap4/4(taps)
  pol1_in9_tap4/1(dout) -> pol1_in9_tap5/1(din)
  pol1_in9_tap4/2(sync_out) -> pol1_in9_tap5/2(sync)
  pol1_in9_tap4/3(coeff_out) -> pol1_in9_tap5/3(coeff)
  pol1_in9_tap4/4(taps_out) -> pol1_in9_tap5/4(taps)
  pol1_in9_tap5/1(dout) -> pol1_in9_tap6/1(din)
  pol1_in9_tap5/2(sync_out) -> pol1_in9_tap6/2(sync)
  pol1_in9_tap5/3(coeff_out) -> pol1_in9_tap6/3(coeff)
  pol1_in9_tap5/4(taps_out) -> pol1_in9_tap6/4(taps)
  pol1_in9_tap6/1(dout) -> pol1_in9_tap7/1(din)
  pol1_in9_tap6/2(sync_out) -> pol1_in9_tap7/2(sync)
  pol1_in9_tap6/3(coeff_out) -> pol1_in9_tap7/3(coeff)
  pol1_in9_tap6/4(taps_out) -> pol1_in9_tap7/4(taps)
  pol1_in9_tap7/1(dout) -> pol1_in9_last_tap/1(din)
  pol1_in9_tap7/2(sync_out) -> pol1_in9_last_tap/2(sync)
  pol1_in9_tap7/3(coeff_out) -> pol1_in9_last_tap/3(coeff)
  pol1_in9_tap7/4(taps_out) -> pol1_in9_last_tap/4(taps)
  pol1_in10/1 -> pol1_in10_coeffs/1(din)
  pol1_in10_coeffs/1(dout) -> pol1_in10_first_tap/1(din)
  pol1_in10_coeffs/3(coeff) -> pol1_in10_first_tap/3(coeffs)
  pol1_in10_first_tap/1(dout) -> pol1_in10_tap2/1(din)
  pol1_in10_first_tap/2(sync_out) -> pol1_in10_tap2/2(sync)
  pol1_in10_first_tap/3(coeff_out) -> pol1_in10_tap2/3(coeff)
  pol1_in10_first_tap/4(taps_out) -> pol1_in10_tap2/4(taps)
  pol1_in10_tap2/1(dout) -> pol1_in10_tap3/1(din)
  pol1_in10_tap2/2(sync_out) -> pol1_in10_tap3/2(sync)
  pol1_in10_tap2/3(coeff_out) -> pol1_in10_tap3/3(coeff)
  pol1_in10_tap2/4(taps_out) -> pol1_in10_tap3/4(taps)
  pol1_in10_tap3/1(dout) -> pol1_in10_tap4/1(din)
  pol1_in10_tap3/2(sync_out) -> pol1_in10_tap4/2(sync)
  pol1_in10_tap3/3(coeff_out) -> pol1_in10_tap4/3(coeff)
  pol1_in10_tap3/4(taps_out) -> pol1_in10_tap4/4(taps)
  pol1_in10_tap4/1(dout) -> pol1_in10_tap5/1(din)
  pol1_in10_tap4/2(sync_out) -> pol1_in10_tap5/2(sync)
  pol1_in10_tap4/3(coeff_out) -> pol1_in10_tap5/3(coeff)
  pol1_in10_tap4/4(taps_out) -> pol1_in10_tap5/4(taps)
  pol1_in10_tap5/1(dout) -> pol1_in10_tap6/1(din)
  pol1_in10_tap5/2(sync_out) -> pol1_in10_tap6/2(sync)
  pol1_in10_tap5/3(coeff_out) -> pol1_in10_tap6/3(coeff)
  pol1_in10_tap5/4(taps_out) -> pol1_in10_tap6/4(taps)
  pol1_in10_tap6/1(dout) -> pol1_in10_tap7/1(din)
  pol1_in10_tap6/2(sync_out) -> pol1_in10_tap7/2(sync)
  pol1_in10_tap6/3(coeff_out) -> pol1_in10_tap7/3(coeff)
  pol1_in10_tap6/4(taps_out) -> pol1_in10_tap7/4(taps)
  pol1_in10_tap7/1(dout) -> pol1_in10_last_tap/1(din)
  pol1_in10_tap7/2(sync_out) -> pol1_in10_last_tap/2(sync)
  pol1_in10_tap7/3(coeff_out) -> pol1_in10_last_tap/3(coeff)
  pol1_in10_tap7/4(taps_out) -> pol1_in10_last_tap/4(taps)
  pol1_in11/1 -> pol1_in11_coeffs/1(din)
  pol1_in11_coeffs/1(dout) -> pol1_in11_first_tap/1(din)
  pol1_in11_coeffs/3(coeff) -> pol1_in11_first_tap/3(coeffs)
  pol1_in11_first_tap/1(dout) -> pol1_in11_tap2/1(din)
  pol1_in11_first_tap/2(sync_out) -> pol1_in11_tap2/2(sync)
  pol1_in11_first_tap/3(coeff_out) -> pol1_in11_tap2/3(coeff)
  pol1_in11_first_tap/4(taps_out) -> pol1_in11_tap2/4(taps)
  pol1_in11_tap2/1(dout) -> pol1_in11_tap3/1(din)
  pol1_in11_tap2/2(sync_out) -> pol1_in11_tap3/2(sync)
  pol1_in11_tap2/3(coeff_out) -> pol1_in11_tap3/3(coeff)
  pol1_in11_tap2/4(taps_out) -> pol1_in11_tap3/4(taps)
  pol1_in11_tap3/1(dout) -> pol1_in11_tap4/1(din)
  pol1_in11_tap3/2(sync_out) -> pol1_in11_tap4/2(sync)
  pol1_in11_tap3/3(coeff_out) -> pol1_in11_tap4/3(coeff)
  pol1_in11_tap3/4(taps_out) -> pol1_in11_tap4/4(taps)
  pol1_in11_tap4/1(dout) -> pol1_in11_tap5/1(din)
  pol1_in11_tap4/2(sync_out) -> pol1_in11_tap5/2(sync)
  pol1_in11_tap4/3(coeff_out) -> pol1_in11_tap5/3(coeff)
  pol1_in11_tap4/4(taps_out) -> pol1_in11_tap5/4(taps)
  pol1_in11_tap5/1(dout) -> pol1_in11_tap6/1(din)
  pol1_in11_tap5/2(sync_out) -> pol1_in11_tap6/2(sync)
  pol1_in11_tap5/3(coeff_out) -> pol1_in11_tap6/3(coeff)
  pol1_in11_tap5/4(taps_out) -> pol1_in11_tap6/4(taps)
  pol1_in11_tap6/1(dout) -> pol1_in11_tap7/1(din)
  pol1_in11_tap6/2(sync_out) -> pol1_in11_tap7/2(sync)
  pol1_in11_tap6/3(coeff_out) -> pol1_in11_tap7/3(coeff)
  pol1_in11_tap6/4(taps_out) -> pol1_in11_tap7/4(taps)
  pol1_in11_tap7/1(dout) -> pol1_in11_last_tap/1(din)
  pol1_in11_tap7/2(sync_out) -> pol1_in11_last_tap/2(sync)
  pol1_in11_tap7/3(coeff_out) -> pol1_in11_last_tap/3(coeff)
  pol1_in11_tap7/4(taps_out) -> pol1_in11_last_tap/4(taps)
  pol1_in12/1 -> pol1_in12_coeffs/1(din)
  pol1_in12_coeffs/1(dout) -> pol1_in12_first_tap/1(din)
  pol1_in12_coeffs/3(coeff) -> pol1_in12_first_tap/3(coeffs)
  pol1_in12_first_tap/1(dout) -> pol1_in12_tap2/1(din)
  pol1_in12_first_tap/2(sync_out) -> pol1_in12_tap2/2(sync)
  pol1_in12_first_tap/3(coeff_out) -> pol1_in12_tap2/3(coeff)
  pol1_in12_first_tap/4(taps_out) -> pol1_in12_tap2/4(taps)
  pol1_in12_tap2/1(dout) -> pol1_in12_tap3/1(din)
  pol1_in12_tap2/2(sync_out) -> pol1_in12_tap3/2(sync)
  pol1_in12_tap2/3(coeff_out) -> pol1_in12_tap3/3(coeff)
  pol1_in12_tap2/4(taps_out) -> pol1_in12_tap3/4(taps)
  pol1_in12_tap3/1(dout) -> pol1_in12_tap4/1(din)
  pol1_in12_tap3/2(sync_out) -> pol1_in12_tap4/2(sync)
  pol1_in12_tap3/3(coeff_out) -> pol1_in12_tap4/3(coeff)
  pol1_in12_tap3/4(taps_out) -> pol1_in12_tap4/4(taps)
  pol1_in12_tap4/1(dout) -> pol1_in12_tap5/1(din)
  pol1_in12_tap4/2(sync_out) -> pol1_in12_tap5/2(sync)
  pol1_in12_tap4/3(coeff_out) -> pol1_in12_tap5/3(coeff)
  pol1_in12_tap4/4(taps_out) -> pol1_in12_tap5/4(taps)
  pol1_in12_tap5/1(dout) -> pol1_in12_tap6/1(din)
  pol1_in12_tap5/2(sync_out) -> pol1_in12_tap6/2(sync)
  pol1_in12_tap5/3(coeff_out) -> pol1_in12_tap6/3(coeff)
  pol1_in12_tap5/4(taps_out) -> pol1_in12_tap6/4(taps)
  pol1_in12_tap6/1(dout) -> pol1_in12_tap7/1(din)
  pol1_in12_tap6/2(sync_out) -> pol1_in12_tap7/2(sync)
  pol1_in12_tap6/3(coeff_out) -> pol1_in12_tap7/3(coeff)
  pol1_in12_tap6/4(taps_out) -> pol1_in12_tap7/4(taps)
  pol1_in12_tap7/1(dout) -> pol1_in12_last_tap/1(din)
  pol1_in12_tap7/2(sync_out) -> pol1_in12_last_tap/2(sync)
  pol1_in12_tap7/3(coeff_out) -> pol1_in12_last_tap/3(coeff)
  pol1_in12_tap7/4(taps_out) -> pol1_in12_last_tap/4(taps)
  pol1_in13/1 -> pol1_in13_coeffs/1(din)
  pol1_in13_coeffs/1(dout) -> pol1_in13_first_tap/1(din)
  pol1_in13_coeffs/3(coeff) -> pol1_in13_first_tap/3(coeffs)
  pol1_in13_first_tap/1(dout) -> pol1_in13_tap2/1(din)
  pol1_in13_first_tap/2(sync_out) -> pol1_in13_tap2/2(sync)
  pol1_in13_first_tap/3(coeff_out) -> pol1_in13_tap2/3(coeff)
  pol1_in13_first_tap/4(taps_out) -> pol1_in13_tap2/4(taps)
  pol1_in13_tap2/1(dout) -> pol1_in13_tap3/1(din)
  pol1_in13_tap2/2(sync_out) -> pol1_in13_tap3/2(sync)
  pol1_in13_tap2/3(coeff_out) -> pol1_in13_tap3/3(coeff)
  pol1_in13_tap2/4(taps_out) -> pol1_in13_tap3/4(taps)
  pol1_in13_tap3/1(dout) -> pol1_in13_tap4/1(din)
  pol1_in13_tap3/2(sync_out) -> pol1_in13_tap4/2(sync)
  pol1_in13_tap3/3(coeff_out) -> pol1_in13_tap4/3(coeff)
  pol1_in13_tap3/4(taps_out) -> pol1_in13_tap4/4(taps)
  pol1_in13_tap4/1(dout) -> pol1_in13_tap5/1(din)
  pol1_in13_tap4/2(sync_out) -> pol1_in13_tap5/2(sync)
  pol1_in13_tap4/3(coeff_out) -> pol1_in13_tap5/3(coeff)
  pol1_in13_tap4/4(taps_out) -> pol1_in13_tap5/4(taps)
  pol1_in13_tap5/1(dout) -> pol1_in13_tap6/1(din)
  pol1_in13_tap5/2(sync_out) -> pol1_in13_tap6/2(sync)
  pol1_in13_tap5/3(coeff_out) -> pol1_in13_tap6/3(coeff)
  pol1_in13_tap5/4(taps_out) -> pol1_in13_tap6/4(taps)
  pol1_in13_tap6/1(dout) -> pol1_in13_tap7/1(din)
  pol1_in13_tap6/2(sync_out) -> pol1_in13_tap7/2(sync)
  pol1_in13_tap6/3(coeff_out) -> pol1_in13_tap7/3(coeff)
  pol1_in13_tap6/4(taps_out) -> pol1_in13_tap7/4(taps)
  pol1_in13_tap7/1(dout) -> pol1_in13_last_tap/1(din)
  pol1_in13_tap7/2(sync_out) -> pol1_in13_last_tap/2(sync)
  pol1_in13_tap7/3(coeff_out) -> pol1_in13_last_tap/3(coeff)
  pol1_in13_tap7/4(taps_out) -> pol1_in13_last_tap/4(taps)
  pol1_in14/1 -> pol1_in14_coeffs/1(din)
  pol1_in14_coeffs/1(dout) -> pol1_in14_first_tap/1(din)
  pol1_in14_coeffs/3(coeff) -> pol1_in14_first_tap/3(coeffs)
  pol1_in14_first_tap/1(dout) -> pol1_in14_tap2/1(din)
  pol1_in14_first_tap/2(sync_out) -> pol1_in14_tap2/2(sync)
  pol1_in14_first_tap/3(coeff_out) -> pol1_in14_tap2/3(coeff)
  pol1_in14_first_tap/4(taps_out) -> pol1_in14_tap2/4(taps)
  pol1_in14_tap2/1(dout) -> pol1_in14_tap3/1(din)
  pol1_in14_tap2/2(sync_out) -> pol1_in14_tap3/2(sync)
  pol1_in14_tap2/3(coeff_out) -> pol1_in14_tap3/3(coeff)
  pol1_in14_tap2/4(taps_out) -> pol1_in14_tap3/4(taps)
  pol1_in14_tap3/1(dout) -> pol1_in14_tap4/1(din)
  pol1_in14_tap3/2(sync_out) -> pol1_in14_tap4/2(sync)
  pol1_in14_tap3/3(coeff_out) -> pol1_in14_tap4/3(coeff)
  pol1_in14_tap3/4(taps_out) -> pol1_in14_tap4/4(taps)
  pol1_in14_tap4/1(dout) -> pol1_in14_tap5/1(din)
  pol1_in14_tap4/2(sync_out) -> pol1_in14_tap5/2(sync)
  pol1_in14_tap4/3(coeff_out) -> pol1_in14_tap5/3(coeff)
  pol1_in14_tap4/4(taps_out) -> pol1_in14_tap5/4(taps)
  pol1_in14_tap5/1(dout) -> pol1_in14_tap6/1(din)
  pol1_in14_tap5/2(sync_out) -> pol1_in14_tap6/2(sync)
  pol1_in14_tap5/3(coeff_out) -> pol1_in14_tap6/3(coeff)
  pol1_in14_tap5/4(taps_out) -> pol1_in14_tap6/4(taps)
  pol1_in14_tap6/1(dout) -> pol1_in14_tap7/1(din)
  pol1_in14_tap6/2(sync_out) -> pol1_in14_tap7/2(sync)
  pol1_in14_tap6/3(coeff_out) -> pol1_in14_tap7/3(coeff)
  pol1_in14_tap6/4(taps_out) -> pol1_in14_tap7/4(taps)
  pol1_in14_tap7/1(dout) -> pol1_in14_last_tap/1(din)
  pol1_in14_tap7/2(sync_out) -> pol1_in14_last_tap/2(sync)
  pol1_in14_tap7/3(coeff_out) -> pol1_in14_last_tap/3(coeff)
  pol1_in14_tap7/4(taps_out) -> pol1_in14_last_tap/4(taps)
  pol1_in15/1 -> pol1_in15_coeffs/1(din)
  pol1_in15_coeffs/1(dout) -> pol1_in15_first_tap/1(din)
  pol1_in15_coeffs/3(coeff) -> pol1_in15_first_tap/3(coeffs)
  pol1_in15_first_tap/1(dout) -> pol1_in15_tap2/1(din)
  pol1_in15_first_tap/2(sync_out) -> pol1_in15_tap2/2(sync)
  pol1_in15_first_tap/3(coeff_out) -> pol1_in15_tap2/3(coeff)
  pol1_in15_first_tap/4(taps_out) -> pol1_in15_tap2/4(taps)
  pol1_in15_tap2/1(dout) -> pol1_in15_tap3/1(din)
  pol1_in15_tap2/2(sync_out) -> pol1_in15_tap3/2(sync)
  pol1_in15_tap2/3(coeff_out) -> pol1_in15_tap3/3(coeff)
  pol1_in15_tap2/4(taps_out) -> pol1_in15_tap3/4(taps)
  pol1_in15_tap3/1(dout) -> pol1_in15_tap4/1(din)
  pol1_in15_tap3/2(sync_out) -> pol1_in15_tap4/2(sync)
  pol1_in15_tap3/3(coeff_out) -> pol1_in15_tap4/3(coeff)
  pol1_in15_tap3/4(taps_out) -> pol1_in15_tap4/4(taps)
  pol1_in15_tap4/1(dout) -> pol1_in15_tap5/1(din)
  pol1_in15_tap4/2(sync_out) -> pol1_in15_tap5/2(sync)
  pol1_in15_tap4/3(coeff_out) -> pol1_in15_tap5/3(coeff)
  pol1_in15_tap4/4(taps_out) -> pol1_in15_tap5/4(taps)
  pol1_in15_tap5/1(dout) -> pol1_in15_tap6/1(din)
  pol1_in15_tap5/2(sync_out) -> pol1_in15_tap6/2(sync)
  pol1_in15_tap5/3(coeff_out) -> pol1_in15_tap6/3(coeff)
  pol1_in15_tap5/4(taps_out) -> pol1_in15_tap6/4(taps)
  pol1_in15_tap6/1(dout) -> pol1_in15_tap7/1(din)
  pol1_in15_tap6/2(sync_out) -> pol1_in15_tap7/2(sync)
  pol1_in15_tap6/3(coeff_out) -> pol1_in15_tap7/3(coeff)
  pol1_in15_tap6/4(taps_out) -> pol1_in15_tap7/4(taps)
  pol1_in15_tap7/1(dout) -> pol1_in15_last_tap/1(din)
  pol1_in15_tap7/2(sync_out) -> pol1_in15_last_tap/2(sync)
  pol1_in15_tap7/3(coeff_out) -> pol1_in15_last_tap/3(coeff)
  pol1_in15_tap7/4(taps_out) -> pol1_in15_last_tap/4(taps)
  pol1_in16/1 -> pol1_in16_coeffs/1(din)
  pol1_in16_coeffs/1(dout) -> pol1_in16_first_tap/1(din)
  pol1_in16_coeffs/3(coeff) -> pol1_in16_first_tap/3(coeffs)
  pol1_in16_first_tap/1(dout) -> pol1_in16_tap2/1(din)
  pol1_in16_first_tap/2(sync_out) -> pol1_in16_tap2/2(sync)
  pol1_in16_first_tap/3(coeff_out) -> pol1_in16_tap2/3(coeff)
  pol1_in16_first_tap/4(taps_out) -> pol1_in16_tap2/4(taps)
  pol1_in16_tap2/1(dout) -> pol1_in16_tap3/1(din)
  pol1_in16_tap2/2(sync_out) -> pol1_in16_tap3/2(sync)
  pol1_in16_tap2/3(coeff_out) -> pol1_in16_tap3/3(coeff)
  pol1_in16_tap2/4(taps_out) -> pol1_in16_tap3/4(taps)
  pol1_in16_tap3/1(dout) -> pol1_in16_tap4/1(din)
  pol1_in16_tap3/2(sync_out) -> pol1_in16_tap4/2(sync)
  pol1_in16_tap3/3(coeff_out) -> pol1_in16_tap4/3(coeff)
  pol1_in16_tap3/4(taps_out) -> pol1_in16_tap4/4(taps)
  pol1_in16_tap4/1(dout) -> pol1_in16_tap5/1(din)
  pol1_in16_tap4/2(sync_out) -> pol1_in16_tap5/2(sync)
  pol1_in16_tap4/3(coeff_out) -> pol1_in16_tap5/3(coeff)
  pol1_in16_tap4/4(taps_out) -> pol1_in16_tap5/4(taps)
  pol1_in16_tap5/1(dout) -> pol1_in16_tap6/1(din)
  pol1_in16_tap5/2(sync_out) -> pol1_in16_tap6/2(sync)
  pol1_in16_tap5/3(coeff_out) -> pol1_in16_tap6/3(coeff)
  pol1_in16_tap5/4(taps_out) -> pol1_in16_tap6/4(taps)
  pol1_in16_tap6/1(dout) -> pol1_in16_tap7/1(din)
  pol1_in16_tap6/2(sync_out) -> pol1_in16_tap7/2(sync)
  pol1_in16_tap6/3(coeff_out) -> pol1_in16_tap7/3(coeff)
  pol1_in16_tap6/4(taps_out) -> pol1_in16_tap7/4(taps)
  pol1_in16_tap7/1(dout) -> pol1_in16_last_tap/1(din)
  pol1_in16_tap7/2(sync_out) -> pol1_in16_last_tap/2(sync)
  pol1_in16_tap7/3(coeff_out) -> pol1_in16_last_tap/3(coeff)
  pol1_in16_tap7/4(taps_out) -> pol1_in16_last_tap/4(taps)
  pol1_in1_last_tap/2(dout0) -> pol1_in_bus_create1/1(in1)
  pol1_in1_last_tap/3(dout1) -> pol1_in_bus_create2/1(in1)
  pol1_in2_last_tap/2(dout0) -> pol1_in_bus_create1/2(in2)
  pol1_in2_last_tap/3(dout1) -> pol1_in_bus_create2/2(in2)
  pol1_in3_last_tap/2(dout0) -> pol1_in_bus_create1/3(in3)
  pol1_in3_last_tap/3(dout1) -> pol1_in_bus_create2/3(in3)
  pol1_in4_last_tap/2(dout0) -> pol1_in_bus_create1/4(in4)
  pol1_in4_last_tap/3(dout1) -> pol1_in_bus_create2/4(in4)
  pol1_in5_last_tap/2(dout0) -> pol1_in_bus_create1/5(in5)
  pol1_in5_last_tap/3(dout1) -> pol1_in_bus_create2/5(in5)
  pol1_in6_last_tap/2(dout0) -> pol1_in_bus_create1/6(in6)
  pol1_in6_last_tap/3(dout1) -> pol1_in_bus_create2/6(in6)
  pol1_in7_last_tap/2(dout0) -> pol1_in_bus_create1/7(in7)
  pol1_in7_last_tap/3(dout1) -> pol1_in_bus_create2/7(in7)
  pol1_in8_last_tap/2(dout0) -> pol1_in_bus_create1/8(in8)
  pol1_in8_last_tap/3(dout1) -> pol1_in_bus_create2/8(in8)
  pol1_in9_last_tap/2(dout0) -> pol1_in_bus_create1/9(in9)
  pol1_in9_last_tap/3(dout1) -> pol1_in_bus_create2/9(in9)
  pol1_in10_last_tap/2(dout0) -> pol1_in_bus_create1/10(in10)
  pol1_in10_last_tap/3(dout1) -> pol1_in_bus_create2/10(in10)
  pol1_in11_last_tap/2(dout0) -> pol1_in_bus_create1/11(in11)
  pol1_in11_last_tap/3(dout1) -> pol1_in_bus_create2/11(in11)
  pol1_in12_last_tap/2(dout0) -> pol1_in_bus_create1/12(in12)
  pol1_in12_last_tap/3(dout1) -> pol1_in_bus_create2/12(in12)
  pol1_in13_last_tap/2(dout0) -> pol1_in_bus_create1/13(in13)
  pol1_in13_last_tap/3(dout1) -> pol1_in_bus_create2/13(in13)
  pol1_in14_last_tap/2(dout0) -> pol1_in_bus_create1/14(in14)
  pol1_in14_last_tap/3(dout1) -> pol1_in_bus_create2/14(in14)
  pol1_in15_last_tap/2(dout0) -> pol1_in_bus_create1/15(in15)
  pol1_in15_last_tap/3(dout1) -> pol1_in_bus_create2/15(in15)
  pol1_in16_last_tap/2(dout0) -> pol1_in_bus_create1/16(in16)
  pol1_in16_last_tap/3(dout1) -> pol1_in_bus_create2/16(in16)
  pol1_in16_last_tap/1(sync_out) -> pol1_transpose/1(sync)
  pol1_in_bus_create1/1(bus_out) -> pol1_transpose/2(in0)
  pol1_in_bus_create2/1(bus_out) -> pol1_transpose/3(in1)
  pol1_transpose/2(out0) -> pol1_reord_in_bus_create/1(in1)
  pol1_transpose/3(out1) -> pol1_reord_in_bus_create/2(in2)
  pol1_reord_in_bus_create/1(bus_out) -> pol1_reord/3(din0)
  pol1_transpose/1(sync_out) -> pol1_reord/1(sync)
  always_we/1 -> pol1_reord/2(en)
  pol1_reord/1(sync_out) -> sync_out/1
  pol1_reord/3(dout0) -> pol1_busexp/1(bus_in)
  pol1_busexp/1(msb_out32) -> pol1_out1/1
  pol1_busexp/2(out31) -> pol1_out2/1
  pol1_busexp/3(out30) -> pol1_out3/1
  pol1_busexp/4(out29) -> pol1_out4/1
  pol1_busexp/5(out28) -> pol1_out5/1
  pol1_busexp/6(out27) -> pol1_out6/1
  pol1_busexp/7(out26) -> pol1_out7/1
  pol1_busexp/8(out25) -> pol1_out8/1
  pol1_busexp/9(out24) -> pol1_out9/1
  pol1_busexp/10(out23) -> pol1_out10/1
  pol1_busexp/11(out22) -> pol1_out11/1
  pol1_busexp/12(out21) -> pol1_out12/1
  pol1_busexp/13(out20) -> pol1_out13/1
  pol1_busexp/14(out19) -> pol1_out14/1
  pol1_busexp/15(out18) -> pol1_out15/1
  pol1_busexp/16(out17) -> pol1_out16/1
  pol1_busexp/17(out16) -> pol1_out17/1
  pol1_busexp/18(out15) -> pol1_out18/1
  pol1_busexp/19(out14) -> pol1_out19/1
  pol1_busexp/20(out13) -> pol1_out20/1
  pol1_busexp/21(out12) -> pol1_out21/1
  pol1_busexp/22(out11) -> pol1_out22/1
  pol1_busexp/23(out10) -> pol1_out23/1
  pol1_busexp/24(out9) -> pol1_out24/1
  pol1_busexp/25(out8) -> pol1_out25/1
  pol1_busexp/26(out7) -> pol1_out26/1
  pol1_busexp/27(out6) -> pol1_out27/1
  pol1_busexp/28(out5) -> pol1_out28/1
  pol1_busexp/29(out4) -> pol1_out29/1
  pol1_busexp/30(out3) -> pol1_out30/1
  pol1_busexp/31(out2) -> pol1_out31/1
  pol1_busexp/32(lsb_out1) -> pol1_out32/1
